simulink model "pasp_16ch_ct"  (Simulink 6.2)
settings: Solver=ode45  StartTime=0.0  StopTime=30000  RelTol=1e-3
undefined symbols (not defined in the file or in its folder): iBOB
libraries: xbsIndex_r3 x1479, casper_library x148, xps_library x58
(part 1 of 11)
settings Model: LastModifiedBy=tfiliba
settings DebuggingCC: SolverPrmCheckMsg=warning

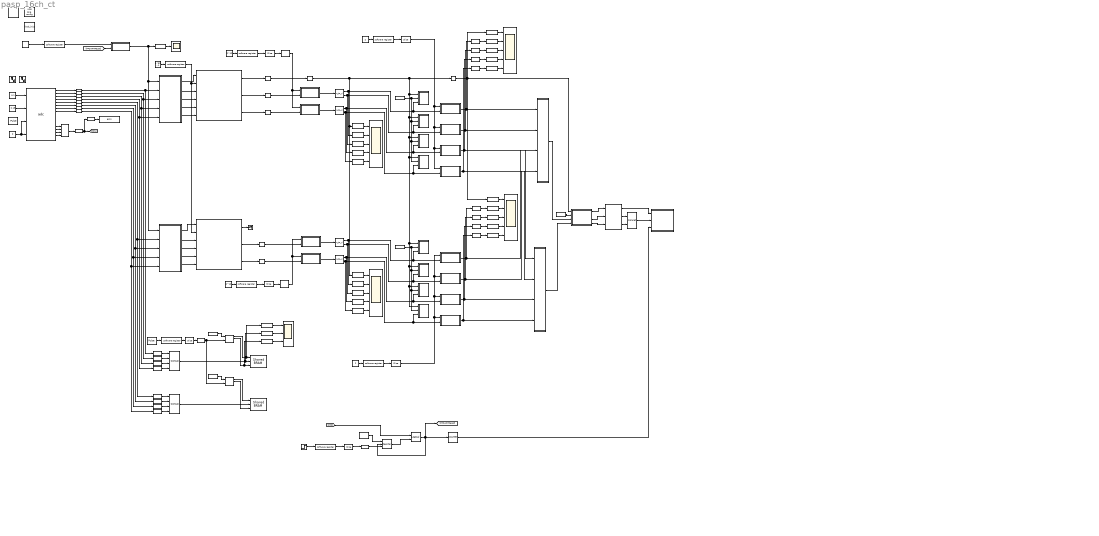
== system pasp_16ch_ct ==
  note: left
  note: Packetized Astronomy Signal Processor
      | Terry Filiba (CASPER)
      | January 2009
      | Version 1.0
  note: n * LCM(reoder_order=2)*(taps*clksperFFT=2*64=128)=256
  note: Pol 1
  note: Pol 2
  note: Real sampling at 800MSa/sec
      | to give B/W of 0-400MHz
  note: ADC Scope
      | Outputs raw bits from ADC so you can measure voltage levels
  note: ARM/PPS Reset Circuit
      | 1. User sets ARM high at half-second
      | 2. 1PPS arrives.
      | 3. PPSARMReset signal goes high for one clock on the 1PPS
      | 4. ARM is reset, and won't go high again until user brings it low then high
  note: Unsigned, 18-bits, b.p. at 12
      | Coefficient by which to scale the output of the FFT.
  note: Selects which 8 bits from 18 are outputted.
      | 0 is lowest 8-bits: bits 0-7 (inclusive)
      | 1: bits 4-9
      | 2: bits 8-15
      | 3 is highest 8-bits: bits 10-17
  note: Extract 8 bits from 18
  note: Extract 8 bits from 18
  note: Delay is here for timing purposes:
      | otherwise adc_sync fails timing.
  " System Generator" : xbsIndex_r3/ System Generator  Tag=genX  xilinxfamily=Virtex2P  part=xc2vp50  speed=-7  package=ff1152  synthesis_tool=XST  directory=./nancay_16ch_ct/sysgen  testbench=off  simulink_period=1  sysclk_period=5  incr_netlist=off  trim_vbits=Everywhere in SubSystem  dbl_ovrd=According to Block Masks  core_generation=According to Block Masks  run_coregen=off  deprecated_control=off  eval_field=0
      settings: AttributesFormatString=System\nGenerator
  Concat1 : xbsIndex_r3/Concat  num_inputs=2  explicit_period=off  period=1  dbl_ovrd=off
  Constant2 : Constant  Value=2
  Constant3 : Constant  Value=2^12
  Constant4 : Constant  Value=2^12
  Constant5 : Constant  Value=2^32 - 1
  Constant6 : Constant  Value=2
  Gateway Out{1..3,8,10..19,21..30} (24 alike) : xbsIndex_r3/Gateway Out  output_type=Double  nbits=8  bin_pt=6  arith_type=Boolean  quantization=Truncate  overflow=Wrap  hdl_port=on  timing_constraint=None  locs_specified=off  LOCs={}  needs_fixed_name=off  show_param=off
      settings: xl_area=[0, 0, 0, 0, 0, 0, 0]
  Reinterpret{,1..3,8..11} (8 alike) : xbsIndex_r3/Reinterpret  force_arith_type=on  arith_type="Signed  (2's comp)"  force_bin_pt=on  bin_pt=0  force_valid=on
  Scope : Scope  NumInputPorts=3
      settings: YMin=-5~-5~-5  YMax=5~5~5
  Scope2 : Scope
      settings: YMin=-1  YMax=1  SaveName=ScopeData2
  Scope{3..6} (4 alike) : Scope  NumInputPorts=5
      Scope3 settings: YMin=-1~-2.5e-005~-1.75e-005~-2.5e-005~-8e-006  YMax=1~0~0~0~0  SaveName=ScopeData3
      Scope4 settings: YMin=-1~-1~-1~-1~-1  YMax=1~0~0~0~0  SaveName=ScopeData4
      Scope5 settings: YMin=-1~-2.5e-005~-1.75e-005~-2.5e-005~-8e-006  YMax=1~0~0~0~0  SaveName=ScopeData5
      Scope6 settings: YMin=-1~-1~-1~-1~-1  YMax=1~0~0~0~0  SaveName=ScopeData6
  Slice10 : xbsIndex_r3/Slice  mode=Lower Bit Location + Width  nbits=2  bit1=0  base1=MSB of Input  bit0=0  base0=LSB of Input  boolean_output=off  explicit_period=off  period=1  dbl_ovrd=off
  Slice2 : xbsIndex_r3/Slice  mode=Lower Bit Location + Width  nbits=2  bit1=0  base1=MSB of Input  bit0=0  base0=LSB of Input  boolean_output=off  explicit_period=off  period=1  dbl_ovrd=off
  Slice3 : xbsIndex_r3/Slice  mode=Lower Bit Location + Width  nbits=18  bit1=0  base1=MSB of Input  bit0=0  base0=LSB of Input  boolean_output=off  explicit_period=off  period=1  dbl_ovrd=off
  Slice4 : xbsIndex_r3/Slice  mode=Lower Bit Location + Width  nbits=18  bit1=0  base1=MSB of Input  bit0=0  base0=LSB of Input  boolean_output=off  explicit_period=off  period=1  dbl_ovrd=off
  Slice8 : xbsIndex_r3/Slice  mode=Lower Bit Location + Width  nbits=1  bit1=0  base1=MSB of Input  bit0=0  base0=LSB of Input  boolean_output=on  explicit_period=off  period=1  dbl_ovrd=off
  Terminator : Terminator
  XSG core config : xps_library/XSG core config  Tag=xps:xsg  hw_sys=iBOB  ibob_linux=off  clk_src=adc1_clk  gpio_clk_io_group=iBOB:sma  gpio_clk_bit_index=0  clk_rate=200  sample_period=1  synthesis_tool=XST  mpc_type=powerpc405
  adc : xps_library/adc  Tag=xps:adc  adc_brd=iBOB:adc1  adc_clk_rate=800  adc_interleave=off  sample_period=1
  adc_data_delay{1..8} (8 alike) : xbsIndex_r3/Delay  latency=1  reg_retiming=on  explicit_period=off  period=1  en=off  accept_only_valid=off  init_zero=on  dbl_ovrd=off  show_param=off
      settings: xl_area=[0, 0, 0, 0, 0, 0, 0]
  bitselect_1 : Subsystem
  bitselect_2 : Subsystem
  bitselect_3 : Subsystem
  bitselect_4 : Subsystem
  bitselect_5 : Subsystem
  bitselect_6 : Subsystem
  bitselect_7 : Subsystem
  bitselect_8 : Subsystem
  bram_adcscope_1 : xps_library/Shared BRAM  Tag=xps:bram  arith_type="Signed  (2's comp)"  addr_width=11  data_width=32  data_bin_pt=0  init_vals=[1:2^11]  sample_rate=1
  bram_adcscope_2 : xps_library/Shared BRAM  Tag=xps:bram  arith_type="Signed  (2's comp)"  addr_width=11  data_width=32  data_bin_pt=0  init_vals=[1:2^11]  sample_rate=1
  bs_delay : xbsIndex_r3/Delay  latency=1  reg_retiming=off  explicit_period=off  period=1  en=off  accept_only_valid=off  init_zero=on  dbl_ovrd=off  show_param=off
      settings: xl_area=[0, 0, 0, 0, 0, 0, 0]
  c_to_ri{1..4} (4 alike) : casper_library/Misc/c_to_ri  n_bits=18  bin_pt=17
      settings: AttributesFormatString=18_17 r/i
  cns_adcscope_1 : xbsIndex_r3/Constant  const=1  equ=P=C  arith_type=Boolean  n_bits=1  bin_pt=0  opselect=C  inp2=PCIN>>17  opr=+  inp1=P  carry=CIN  iostate=0  explicit_period=on  period=1  dbl_ovrd=off
  cns_adcscope_2 : xbsIndex_r3/Constant  const=1  equ=P=C  arith_type=Boolean  n_bits=1  bin_pt=0  opselect=C  inp2=PCIN>>17  opr=+  inp1=P  carry=CIN  iostate=0  explicit_period=on  period=1  dbl_ovrd=off
  cns_reset : xbsIndex_r3/Constant  const=1  equ=P=C  arith_type=Boolean  n_bits=1  bin_pt=0  opselect=C  inp2=PCIN>>17  opr=+  inp1=P  carry=CIN  iostate=0  explicit_period=on  period=1  dbl_ovrd=off
  cns_scopes_en0 : xbsIndex_r3/Constant  const=1  equ=P=C  arith_type=Boolean  n_bits=1  bin_pt=0  opselect=C  inp2=PCIN>>17  opr=+  inp1=P  carry=CIN  iostate=0  explicit_period=on  period=1  dbl_ovrd=off
  cns_scopes_en1 : xbsIndex_r3/Constant  const=1  equ=P=C  arith_type=Boolean  n_bits=1  bin_pt=0  opselect=C  inp2=PCIN>>17  opr=+  inp1=P  carry=CIN  iostate=0  explicit_period=on  period=1  dbl_ovrd=off
  cns_sync_period : Constant  Value=10240
  cns_trotfrt_rnf2 : xbsIndex_r3/Constant  const=1  equ=P=C  arith_type=Boolean  n_bits=1  bin_pt=0  opselect=C  inp2=PCIN>>17  opr=+  inp1=P  carry=CIN  iostate=0  explicit_period=on  period=1  dbl_ovrd=off
  cnt_adcscope_1 : casper_library/Misc/freeze_cntr  CounterBits=11
  cnt_adcscope_2 : casper_library/Misc/freeze_cntr  CounterBits=11
  coeff_delay : xbsIndex_r3/Delay  latency=6  reg_retiming=on  explicit_period=off  period=1  en=off  accept_only_valid=off  init_zero=on  dbl_ovrd=off  show_param=off
      settings: xl_area=[0, 0, 0, 0, 0, 0, 0]
  concat_adcscope_1 : xbsIndex_r3/Concat  num_inputs=4  explicit_period=off  period=1  dbl_ovrd=off
  concat_adcscope_2 : xbsIndex_r3/Concat  num_inputs=4  explicit_period=off  period=1  dbl_ovrd=off
  cram0 : Subsystem  AncestorBlock=gavrt_library/cram  mask(cram){num_slice=4}
      mask prompts: num_slice "Number of slices"
      mask help: Concatenates inputs together after forcing binary point to zero.
      mask init:
      | cram_init(gcb, ...
      |     'num_slice', num_slice);
  cram1 : Subsystem  AncestorBlock=gavrt_library/cram  mask(cram){num_slice=4}
      mask prompts: num_slice "Number of slices"
      mask help: Concatenates inputs together after forcing binary point to zero.
      mask init:
      | cram_init(gcb, ...
      |     'num_slice', num_slice);
  dist_gbe : Subsystem  mask(dist_gbe){numcomputers=16, numsamples=16, samplesperpacket=64}
      mask prompts: numcomputers "Num IPs (Must be power of 2)"; numsamples "Samples per spectrum (Number of clock cycles to generate 1 spectrum)"; samplesperpacket "Samples per packet (Number of samples to put in a packet)"
      mask init:
      | dist_gbe_init(gcb,...
      |     'numcomputers', numcomputers,...
      |     'numsamples', numsamples,...
      |     'samplesperpacket', samplesperpacket)
      settings: AttributesFormatString=IPs=16
  fft_delay : xbsIndex_r3/Delay  latency=4  reg_retiming=off  explicit_period=off  period=1  en=off  accept_only_valid=off  init_zero=on  dbl_ovrd=off  show_param=off
      settings: xl_area=[0, 0, 0, 0, 0, 0, 0]
  fft_wideband_real : Subsystem  AncestorBlock=casper_library/FFTs/fft_wideband_real  mask(fft_wideband_real){FFTSize=5, BitWidth=18, n_inputs=2, quantization=Truncate, overflow=Wrap, add_latency=2, mult_latency=3, bram_latency=2}
      mask prompts: FFTSize "Size of FFT: (2^?)"; BitWidth "Bit Width"; n_inputs "Number of Simultaneous Inputs: (2^?)"; quantization "Quantization Behavior"; overflow "Overflow Behavior"; add_latency "Add Latency"; mult_latency "Mult Latency"; bram_latency "BRAM Latency"
      mask init:
      | fft_wideband_real_init(gcb,...
      |     'FFTSize', FFTSize,...
      |     'BitWidth', BitWidth,...
      |     'n_inputs', n_inputs,...
      |     'quantization', quantization,...
      |     'overflow', overflow,...
      |     'add_latency', add_latency,...
      |     'mult_latency', mult_latency,...
      |     'bram_latency', bram_latency);
      settings: AttributesFormatString=FFTSize=5, n_inputs=2
      mask StyleString: edit,edit,edit,popup(Truncate|Round  (unbiased: +/- Inf)|Round  (unbiased: Even Values)),popup(Wrap|Saturate|Error),edit,edit,edit
  fft_wideband_real1 : Subsystem  AncestorBlock=casper_library/FFTs/fft_wideband_real  mask(fft_wideband_real){FFTSize=5, BitWidth=18, n_inputs=2, quantization=Truncate, overflow=Wrap, add_latency=2, mult_latency=3, bram_latency=2}
      mask prompts: FFTSize "Size of FFT: (2^?)"; BitWidth "Bit Width"; n_inputs "Number of Simultaneous Inputs: (2^?)"; quantization "Quantization Behavior"; overflow "Overflow Behavior"; add_latency "Add Latency"; mult_latency "Mult Latency"; bram_latency "BRAM Latency"
      mask init: same as pasp_16ch_ct/fft_wideband_real
      settings: AttributesFormatString=FFTSize=5, n_inputs=2
      mask StyleString: edit,edit,edit,popup(Truncate|Round  (unbiased: +/- Inf)|Round  (unbiased: Even Values)),popup(Wrap|Saturate|Error),edit,edit,edit
  fftdata_delay{1..4} (4 alike) : xbsIndex_r3/Delay  latency=4  reg_retiming=on  explicit_period=off  period=1  en=off  accept_only_valid=off  init_zero=on  dbl_ovrd=off  show_param=off
      settings: xl_area=[0, 0, 0, 0, 0, 0, 0]
  force_adc_i{0..7} (8 alike) : xbsIndex_r3/Reinterpret  force_arith_type=on  arith_type=Unsigned  force_bin_pt=on  bin_pt=0  force_valid=on
  ibob_lwip : xps_library/ibob_lwip
  led2_pps : xps_library/gpio  Tag=xps:gpio  io_group=iBOB:led  io_dir=out  arith_type=Boolean  bitwidth=1  bin_pt=0  bit_index=3  sample_period=1  use_single_ended=off  use_ddr=off  reg_iob=on  reg_clk_phase=0  termination=None
  log_arm_pps : xbsIndex_r3/Logical  logical_function=AND  inputs=2  precision=Full  arith_type=Unsigned  n_bits=8  bin_pt=2  align_bp=on  latency=0  explicit_period=off  period=1  en=off  dbl_ovrd=off  show_param=off
      settings: xl_area=[0, 0, 0, 0, 0, 0, 0]
  pfb_fir_real : Subsystem  AncestorBlock=casper_library/PFBs/pfb_fir_real  mask(pfb_fir_real){PFBSize=5, TotalTaps=2, WindowType=hamming, n_inputs=2, MakeBiplex=0, BitWidthIn=8, BitWidthOut=18, CoeffBitWidth=8, CoeffDistMem=1, CoeffRound=0, add_latency=1, mult_latency=2, bram_latency=2, quantization=Truncate, fwidth=1}
      mask prompts: PFBSize "Size of PFB: (2^? pnts)"; TotalTaps "Total Number of Taps:"; WindowType "Windowing Function:"; n_inputs "Number of Simultaneous Inputs: (2^?)"; MakeBiplex "Make Biplex"; BitWidthIn "Input Bitwidth:"; BitWidthOut "Output Bitwidth:"; CoeffBitWidth "Coefficient Bitwidth:"; CoeffDistMem "Use Distributed Memory for Coeffs"; CoeffRound "Round Coefficients"; add_latency "Add Latency"; mult_latency "Mult Latency"; bram_latency "BRAM Latency"; quantization "Quantization Behavior"; fwidth "Bin Width Scaling (normal=1)"
      mask init:
      | pfb_fir_real_init(gcb,...
      |     'PFBSize', PFBSize,...
      |     'TotalTaps', TotalTaps,...
      |     'WindowType', WindowType,...
      |     'n_inputs', n_inputs,...
      |     'MakeBiplex', MakeBiplex,...
      |     'BitWidthIn', BitWidthIn,...
      |     'BitWidthOut', BitWidthOut,...
      |     'CoeffBitWidth', CoeffBitWidth,...
      |     'CoeffDistMem', CoeffDistMem,...
      |     'CoeffRound', CoeffRound,...
      |     'add_latency', add_latency,...
      |     'mult_latency', mult_latency,...
      |     'bram_latency', bram_latency,...
      |     'quantization', quantization,...
      |     'fwidth', fwidth);
      settings: AttributesFormatString=taps=2, add_latency=1
      mask StyleString: edit,edit,popup(bartlett|barthannwin|blackman|blackmanharris|bohamwin|chebwin|flattopwin|gausswin|hamming|hann|kaiser|nuttallwin|parzenwin|rectwin|tukeywin|triang),edit,edit,edit,edit,edit,edit,edit,edit,edit,edit,popup(Truncate|Round  (unbiased: +/- Inf)|Round  (unbiased: Even Values)),edit
  pfb_fir_real1 : Subsystem  AncestorBlock=casper_library/PFBs/pfb_fir_real  mask(pfb_fir_real){PFBSize=5, TotalTaps=3, WindowType=hamming, n_inputs=2, MakeBiplex=0, BitWidthIn=8, BitWidthOut=18, CoeffBitWidth=8, CoeffDistMem=1, CoeffRound=0, add_latency=1, mult_latency=2, bram_latency=2, quantization=Truncate, fwidth=1}
      mask prompts: PFBSize "Size of PFB: (2^? pnts)"; TotalTaps "Total Number of Taps:"; WindowType "Windowing Function:"; n_inputs "Number of Simultaneous Inputs: (2^?)"; MakeBiplex "Make Biplex"; BitWidthIn "Input Bitwidth:"; BitWidthOut "Output Bitwidth:"; CoeffBitWidth "Coefficient Bitwidth:"; CoeffDistMem "Use Distributed Memory for Coeffs"; CoeffRound "Round Coefficients"; add_latency "Add Latency"; mult_latency "Mult Latency"; bram_latency "BRAM Latency"; quantization "Quantization Behavior"; fwidth "Bin Width Scaling (normal=1)"
      mask init: same as pasp_16ch_ct/pfb_fir_real
      settings: AttributesFormatString=taps=3, add_latency=1
      mask StyleString: edit,edit,popup(bartlett|barthannwin|blackman|blackmanharris|bohamwin|chebwin|flattopwin|gausswin|hamming|hann|kaiser|nuttallwin|parzenwin|rectwin|tukeywin|triang),edit,edit,edit,edit,edit,edit,edit,edit,edit,edit,popup(Truncate|Round  (unbiased: +/- Inf)|Round  (unbiased: Even Values)),edit
  posedge_adcscope : casper_library/Misc/posedge  Tag=Rising Edge Detector
  posedge_arm : casper_library/Misc/posedge  Tag=Rising Edge Detector
  posedge_pps : casper_library/Misc/posedge  Tag=Rising Edge Detector
  pulse_ext : casper_library/Misc/pulse_ext  pulse_len=10000000
  reg_adcscope_trigger : xps_library/software register  Tag=xps:sw_reg  io_dir=From Processor  arith_type=Unsigned  bitwidth=32  bin_pt=0  sample_period=1  gw_name=pasp_16ch_ct_reg_adcscope_trigger_user_data_out
  reg_arm : xps_library/software register  Tag=xps:sw_reg  io_dir=From Processor  arith_type=Unsigned  bitwidth=32  bin_pt=0  sample_period=1  gw_name=pasp_16ch_ct_reg_arm_user_data_out
  reg_coeff_pol1 : xps_library/software register  Tag=xps:sw_reg  io_dir=From Processor  arith_type=Unsigned  bitwidth=32  bin_pt=0  sample_period=1  gw_name=pasp_16ch_ct_reg_coeff_pol1_user_data_out
  reg_coeff_pol2 : xps_library/software register  Tag=xps:sw_reg  io_dir=From Processor  arith_type=Unsigned  bitwidth=32  bin_pt=0  sample_period=1  gw_name=pasp_16ch_ct_reg_coeff_pol2_user_data_out
  reg_fft_shift : xps_library/software register  Tag=xps:sw_reg  io_dir=From Processor  arith_type=Unsigned  bitwidth=32  bin_pt=0  sample_period=1  gw_name=pasp_16ch_ct_reg_fft_shift_user_data_out
  reg_output_bitselect_pol1 : xps_library/software register  Tag=xps:sw_reg  io_dir=From Processor  arith_type=Unsigned  bitwidth=32  bin_pt=0  sample_period=1  gw_name=pasp_16ch_ct_reg_output_bitselect_pol1_user_data_out
  reg_output_bitselect_pol2 : xps_library/software register  Tag=xps:sw_reg  io_dir=From Processor  arith_type=Unsigned  bitwidth=32  bin_pt=0  sample_period=1  gw_name=pasp_16ch_ct_reg_output_bitselect_pol2_user_data_out
  reg_reset_arm : xbsIndex_r3/Register  init=0  reg_only_valid=off  explicit_period=on  period=1  rst=on  en=on  out_en=off  dbl_ovrd=off  show_param=off
      settings: xl_area=[0, 0, 0, 0, 0, 0, 0]
  reg_sync_period : xps_library/software register  Tag=xps:sw_reg  io_dir=From Processor  arith_type=Unsigned  bitwidth=32  bin_pt=0  sample_period=1  gw_name=pasp_16ch_ct_reg_sync_period_user_data_out
  reint : xbsIndex_r3/Reinterpret  force_arith_type=on  arith_type=Unsigned  force_bin_pt=on  bin_pt=12  force_valid=on
  reint1 : xbsIndex_r3/Reinterpret  force_arith_type=on  arith_type=Unsigned  force_bin_pt=on  bin_pt=12  force_valid=on
  reorder : Subsystem  AncestorBlock=casper_library/Reorder/reorder  mask(reorder){map=[0 8 1 9 2 10 3 11 4 12 5 13 6 14 7 15], n_inputs=2, bram_latency=2, map_latency=1, double_buffer=0}
      mask prompts: map "Output Order:"; n_inputs "Number of inputs"; bram_latency "BRAM Latency"; map_latency "Map Latency"; double_buffer "Double Buffer"
      mask init:
      | reorder_init(gcb, ...
      |     'map', map, ...
      |     'n_inputs', n_inputs, ...
      |     'bram_latency', bram_latency, ...
      |     'map_latency', map_latency, ...
      |     'double_buffer', double_buffer);
      settings: AttributesFormatString=order=4
  scale1 : Subsystem
  scale2 : Subsystem
  scale3 : Subsystem
  scale4 : Subsystem
  scope_output1 : Subsystem
  scope_output2 : Subsystem
  scope_output3 : Subsystem
  scope_output4 : Subsystem
  scope_output5 : Subsystem
  scope_output6 : Subsystem
  scope_output7 : Subsystem
  scope_output8 : Subsystem
  sim_1pps : DiscretePulseGenerator  Period=1000  PulseWidth=3
  sim_adcscope_trigger : DiscretePulseGenerator  Period=5000
  sim_cns : Constant  Value=0.1
  sim_cns1 : Constant  Value=0.15
  sim_sine : Sin  Amplitude=0.8  Frequency=2 * pi * (256/1024)  Samples=0.12566  SampleTime=1/4
  sim_sine1 : Sin  Amplitude=0.8  Frequency=2 * pi * (128/1024)  Samples=0.12566  SampleTime=1/4
  sim_step_arm : Step  SampleTime=0
  sim_zero : Constant  Value=0
  slc_arm : xbsIndex_r3/Slice  mode=Lower Bit Location + Width  nbits=1  bit1=0  base1=MSB of Input  bit0=0  base0=LSB of Input  boolean_output=on  explicit_period=off  period=1  dbl_ovrd=off
  square_transposer : casper_library/Reorder/square_transposer  n_inputs=1
      settings: AttributesFormatString=n_inputs=1
  sync_generator : Subsystem
  sync_or : xbsIndex_r3/Logical  logical_function=OR  inputs=4  precision=Full  arith_type=Unsigned  n_bits=8  bin_pt=2  align_bp=on  latency=1  explicit_period=off  period=1  en=off  dbl_ovrd=off  show_param=off
      settings: xl_area=[0, 0, 0, 0, 0, 0, 0]
  system_counter : xbsIndex_r3/Counter  cnt_type=Free Running  n_bits=64  bin_pt=0  arith_type=Unsigned  start_count=0  cnt_to=Inf  cnt_by_val=1  operation=Up  explicit_period=off  period=1  load_pin=off  rst=on  en=off  dbl_ovrd=off  show_param=off  use_rpm=on  gen_core=off
      settings: xl_area=[0, 0, 0, 0, 0, 0, 0]
  wires:
  reg_fft_shift/1 -> fft_wideband_real/2(shift), fft_wideband_real1/2(shift)
  fft_wideband_real/1(sync_out) -> fft_delay/1
  fft_wideband_real1/1(sync_out) -> Terminator/1
  reg_sync_period/1 -> sync_generator/1(period)
  sim_zero/1 -> adc/4, adc/3
  adc/1 -> adc_data_delay1/1
  sync_generator/1(sync) -> Gateway Out8/1, pfb_fir_real/1(sync), pfb_fir_real1/1(sync)
  adc/2 -> adc_data_delay2/1
  adc/3 -> adc_data_delay3/1
  adc/4 -> adc_data_delay4/1
  adc/5 -> adc_data_delay5/1
  adc/6 -> adc_data_delay6/1
  adc/7 -> adc_data_delay7/1
  adc/8 -> adc_data_delay8/1
  cns_sync_period/1 -> reg_sync_period/1
  adc/13 -> sync_or/1
  adc/14 -> sync_or/2
  adc/15 -> sync_or/3
  adc/16 -> sync_or/4
  sync_or/1 -> posedge_pps/1
  Gateway Out8/1 -> Scope2/1
  posedge_pps/1 -> [PPS], pulse_ext/1
  [PPSARMReset] -> sync_generator/2(reset)
  pulse_ext/1 -> led2_pps/1
  reg_arm/1 -> slc_arm/1
  cns_reset/1 -> reg_reset_arm/1
  reg_reset_arm/1 -> log_arm_pps/2
  [PPS] -> log_arm_pps/1
  log_arm_pps/1 -> reg_reset_arm/2, system_counter/1, [PPSARMReset]
  slc_arm/1 -> posedge_arm/1
  posedge_arm/1 -> reg_reset_arm/3
  concat_adcscope_1/1 -> bram_adcscope_1/2, Gateway Out2/1
  force_adc_i0/1 -> concat_adcscope_1/1
  force_adc_i1/1 -> concat_adcscope_1/2
  force_adc_i2/1 -> concat_adcscope_1/3
  force_adc_i3/1 -> concat_adcscope_1/4
  force_adc_i4/1 -> concat_adcscope_2/1
  force_adc_i5/1 -> concat_adcscope_2/2
  force_adc_i6/1 -> concat_adcscope_2/3
  force_adc_i7/1 -> concat_adcscope_2/4
  sim_step_arm/1 -> reg_arm/1
  Constant3/1 -> reg_coeff_pol1/1
  reg_coeff_pol1/1 -> Slice3/1
  fft_wideband_real/2(out0) -> fftdata_delay1/1
  Slice3/1 -> reint/1
  coeff_delay/1 -> scope_output1/1(rst), scope_output2/1(rst), scope_output3/1(rst), scope_output5/1(rst), scope_output6/1(rst), scope_output7/1(rst), scope_output8/1(rst), scope_output4/1(rst), bs_delay/1, Gateway Out11/1, Gateway Out22/1
  scale1/1(data_out) -> c_to_ri1/1
  reint/1 -> scale1/1(coeff), scale2/1(coeff)
  scale2/1(data_out) -> c_to_ri2/1
  fft_wideband_real/3(out1) -> fftdata_delay2/1
  fft_wideband_real1/2(out0) -> fftdata_delay3/1
  fft_wideband_real1/3(out1) -> fftdata_delay4/1
  Constant4/1 -> reg_coeff_pol2/1
  reg_coeff_pol2/1 -> Slice4/1
  Slice4/1 -> reint1/1
  reint1/1 -> scale3/1(coeff), scale4/1(coeff)
  Constant2/1 -> reg_output_bitselect_pol1/1
  reg_output_bitselect_pol1/1 -> Slice2/1
  c_to_ri1/1 -> bitselect_1/2(data_in), scope_output1/3(data_in), Gateway Out12/1
  c_to_ri2/2 -> Gateway Out14/1, bitselect_4/2(data_in), scope_output4/3(data_in)
  c_to_ri2/1 -> Gateway Out13/1, bitselect_3/2(data_in), scope_output3/3(data_in)
  c_to_ri1/2 -> scope_output2/3(data_in), bitselect_2/2(data_in), Gateway Out10/1
  bitselect_1/1(data_out) -> cram0/1(In1), Reinterpret/1
  bitselect_2/1(data_out) -> cram0/2(In2), Reinterpret1/1
  bitselect_3/1(data_out) -> Reinterpret2/1, cram1/1(In1)
  bitselect_4/1(data_out) -> Reinterpret3/1, cram1/2(In2)
  Constant5/1 -> reg_fft_shift/1
  cnt_adcscope_1/1 -> bram_adcscope_1/1, Gateway Out1/1
  cnt_adcscope_1/2 -> bram_adcscope_1/3, Gateway Out3/1
  cns_adcscope_1/1 -> cnt_adcscope_1/1
  sim_adcscope_trigger/1 -> reg_adcscope_trigger/1
  reg_adcscope_trigger/1 -> Slice8/1
  posedge_adcscope/1 -> cnt_adcscope_1/2, cnt_adcscope_2/2
  concat_adcscope_2/1 -> bram_adcscope_2/2
  cnt_adcscope_2/1 -> bram_adcscope_2/1
  cnt_adcscope_2/2 -> bram_adcscope_2/3
  cns_adcscope_2/1 -> cnt_adcscope_2/1
  Gateway Out1/1 -> Scope/1
  Gateway Out2/1 -> Scope/2
  Gateway Out3/1 -> Scope/3
  cns_scopes_en0/1 -> scope_output1/2(en), scope_output2/2(en), scope_output3/2(en), scope_output4/2(en)
  Slice2/1 -> bitselect_1/1(bitselect), bitselect_2/1(bitselect), bitselect_3/1(bitselect), bitselect_4/1(bitselect)
  sim_cns/1 -> adc/1
  Gateway Out11/1 -> Scope3/1
  Gateway Out12/1 -> Scope3/2
  Gateway Out10/1 -> Scope3/3
  Gateway Out13/1 -> Scope3/4
  Gateway Out14/1 -> Scope3/5
  bs_delay/1 -> Gateway Out16/1, Gateway Out27/1, reorder/1(sync)
  Gateway Out16/1 -> Scope4/1
  Gateway Out17/1 -> Scope4/2
  Gateway Out15/1 -> Scope4/3
  Gateway Out18/1 -> Scope4/4
  Gateway Out19/1 -> Scope4/5
  Slice8/1 -> posedge_adcscope/1
  Reinterpret/1 -> Gateway Out17/1
  Reinterpret1/1 -> Gateway Out15/1
  Reinterpret2/1 -> Gateway Out18/1
  Reinterpret3/1 -> Gateway Out19/1
  c_to_ri3/1 -> bitselect_5/2(data_in), scope_output5/3(data_in), Gateway Out23/1
  c_to_ri4/2 -> Gateway Out25/1, bitselect_8/2(data_in), scope_output8/3(data_in)
  c_to_ri4/1 -> Gateway Out24/1, bitselect_7/2(data_in), scope_output7/3(data_in)
  c_to_ri3/2 -> scope_output6/3(data_in), bitselect_6/2(data_in), Gateway Out21/1
  bitselect_5/1(data_out) -> Reinterpret8/1, cram0/3(In3)
  bitselect_6/1(data_out) -> Reinterpret9/1, cram0/4(In4)
  bitselect_7/1(data_out) -> cram1/3(In3), Reinterpret10/1
  bitselect_8/1(data_out) -> cram1/4(In4), Reinterpret11/1
  cns_scopes_en1/1 -> scope_output5/2(en), scope_output6/2(en), scope_output7/2(en), scope_output8/2(en)
  Gateway Out22/1 -> Scope5/1
  Gateway Out23/1 -> Scope5/2
  Gateway Out21/1 -> Scope5/3
  Gateway Out24/1 -> Scope5/4
  Gateway Out25/1 -> Scope5/5
  scale3/1(data_out) -> c_to_ri3/1
  scale4/1(data_out) -> c_to_ri4/1
  Gateway Out27/1 -> Scope6/1
  Gateway Out28/1 -> Scope6/2
  Gateway Out26/1 -> Scope6/3
  Gateway Out29/1 -> Scope6/4
  Gateway Out30/1 -> Scope6/5
  Reinterpret8/1 -> Gateway Out28/1
  Reinterpret9/1 -> Gateway Out26/1
  Reinterpret10/1 -> Gateway Out29/1
  Reinterpret11/1 -> Gateway Out30/1
  sim_cns1/1 -> adc/2
  Constant6/1 -> reg_output_bitselect_pol2/1
  reg_output_bitselect_pol2/1 -> Slice10/1
  Slice10/1 -> bitselect_5/1(bitselect), bitselect_6/1(bitselect), bitselect_7/1(bitselect), bitselect_8/1(bitselect)
  pfb_fir_real/2(pol1_out1) -> fft_wideband_real/3(in0)
  pfb_fir_real/3(pol1_out2) -> fft_wideband_real/4(in1)
  pfb_fir_real/4(pol1_out3) -> fft_wideband_real/5(in2)
  pfb_fir_real/5(pol1_out4) -> fft_wideband_real/6(in3)
  pfb_fir_real1/2(pol1_out1) -> fft_wideband_real1/3(in0)
  pfb_fir_real1/3(pol1_out2) -> fft_wideband_real1/4(in1)
  pfb_fir_real1/4(pol1_out3) -> fft_wideband_real1/5(in2)
  pfb_fir_real1/5(pol1_out4) -> fft_wideband_real1/6(in3)
  pfb_fir_real/1(sync_out) -> fft_wideband_real/1(sync)
  pfb_fir_real1/1(sync_out) -> fft_wideband_real1/1(sync)
  fft_delay/1 -> coeff_delay/1
  fftdata_delay1/1 -> scale1/2(data_in)
  fftdata_delay2/1 -> scale2/2(data_in)
  fftdata_delay3/1 -> scale3/2(data_in)
  fftdata_delay4/1 -> scale4/2(data_in)
  adc_data_delay1/1 -> force_adc_i0/1, pfb_fir_real/2(pol1_in1)
  adc_data_delay2/1 -> force_adc_i1/1, pfb_fir_real/3(pol1_in2)
  adc_data_delay3/1 -> force_adc_i2/1, pfb_fir_real/4(pol1_in3)
  adc_data_delay4/1 -> force_adc_i3/1, pfb_fir_real/5(pol1_in4)
  adc_data_delay5/1 -> force_adc_i4/1, pfb_fir_real1/2(pol1_in1)
  adc_data_delay6/1 -> force_adc_i5/1, pfb_fir_real1/3(pol1_in2)
  adc_data_delay7/1 -> force_adc_i6/1, pfb_fir_real1/4(pol1_in3)
  adc_data_delay8/1 -> force_adc_i7/1, pfb_fir_real1/5(pol1_in4)
  system_counter/1 -> dist_gbe/3(sys_counter)
  square_transposer/1 -> dist_gbe/1(sync)
  square_transposer/2 -> Concat1/1
  square_transposer/3 -> Concat1/2
  Concat1/1 -> dist_gbe/2(data_in)
  reorder/1(sync_out) -> square_transposer/1
  reorder/3(dout0) -> square_transposer/2
  reorder/4(dout1) -> square_transposer/3
  cns_trotfrt_rnf2/1 -> reorder/2(en)
  cram0/1(Out) -> reorder/3(din0)
  cram1/1(Out) -> reorder/4(din1)

== system pasp_16ch_ct/bitselect_1 ==
  bitselect : Inport  Port=1  LatchInput=off
  data_in : Inport  Port=2  LatchInput=off
  mux_bitselect : xbsIndex_r3/Mux  inputs=4  precision=Full  arith_type="Signed  (2's comp)"  n_bits=8  bin_pt=2  quantization=Truncate  overflow=Wrap  latency=1  explicit_period=off  period=1  en=off  dbl_ovrd=off  show_param=off  mux_type=off  use_rpm=off  gen_core=off
      settings: xl_area=[0, 0, 0, 0, 0, 0, 0]
  reint_bp_0 : xbsIndex_r3/Reinterpret  force_arith_type=on  arith_type=Unsigned  force_bin_pt=on  bin_pt=0  force_valid=on
  slc_bitselect_1 : xbsIndex_r3/Slice  mode=Lower Bit Location + Width  nbits=8  bit1=0  base1=MSB of Input  bit0=0  base0=LSB of Input  boolean_output=off  explicit_period=off  period=1  dbl_ovrd=off
  slc_bitselect_2 : xbsIndex_r3/Slice  mode=Lower Bit Location + Width  nbits=8  bit1=0  base1=MSB of Input  bit0=4  base0=LSB of Input  boolean_output=off  explicit_period=off  period=1  dbl_ovrd=off
  slc_bitselect_3 : xbsIndex_r3/Slice  mode=Lower Bit Location + Width  nbits=8  bit1=0  base1=MSB of Input  bit0=8  base0=LSB of Input  boolean_output=off  explicit_period=off  period=1  dbl_ovrd=off
  slc_bitselect_4 : xbsIndex_r3/Slice  mode=Lower Bit Location + Width  nbits=8  bit1=0  base1=MSB of Input  bit0=10  base0=LSB of Input  boolean_output=off  explicit_period=off  period=1  dbl_ovrd=off
  data_out : Outport
  wires:
  slc_bitselect_1/1 -> mux_bitselect/2
  slc_bitselect_2/1 -> mux_bitselect/3
  slc_bitselect_3/1 -> mux_bitselect/4
  slc_bitselect_4/1 -> mux_bitselect/5
  data_in/1 -> reint_bp_0/1
  bitselect/1 -> mux_bitselect/1
  mux_bitselect/1 -> data_out/1
  reint_bp_0/1 -> slc_bitselect_4/1, slc_bitselect_3/1, slc_bitselect_2/1, slc_bitselect_1/1

== system pasp_16ch_ct/bitselect_2 ==
  bitselect : Inport  Port=1  LatchInput=off
  data_in : Inport  Port=2  LatchInput=off
  mux_bitselect : xbsIndex_r3/Mux  inputs=4  precision=Full  arith_type="Signed  (2's comp)"  n_bits=8  bin_pt=2  quantization=Truncate  overflow=Wrap  latency=1  explicit_period=off  period=1  en=off  dbl_ovrd=off  show_param=off  mux_type=off  use_rpm=off  gen_core=off
      settings: xl_area=[0, 0, 0, 0, 0, 0, 0]
  reint_bp_0 : xbsIndex_r3/Reinterpret  force_arith_type=on  arith_type=Unsigned  force_bin_pt=on  bin_pt=0  force_valid=on
  slc_bitselect_1 : xbsIndex_r3/Slice  mode=Lower Bit Location + Width  nbits=8  bit1=0  base1=MSB of Input  bit0=0  base0=LSB of Input  boolean_output=off  explicit_period=off  period=1  dbl_ovrd=off
  slc_bitselect_2 : xbsIndex_r3/Slice  mode=Lower Bit Location + Width  nbits=8  bit1=0  base1=MSB of Input  bit0=4  base0=LSB of Input  boolean_output=off  explicit_period=off  period=1  dbl_ovrd=off
  slc_bitselect_3 : xbsIndex_r3/Slice  mode=Lower Bit Location + Width  nbits=8  bit1=0  base1=MSB of Input  bit0=8  base0=LSB of Input  boolean_output=off  explicit_period=off  period=1  dbl_ovrd=off
  slc_bitselect_4 : xbsIndex_r3/Slice  mode=Lower Bit Location + Width  nbits=8  bit1=0  base1=MSB of Input  bit0=10  base0=LSB of Input  boolean_output=off  explicit_period=off  period=1  dbl_ovrd=off
  data_out : Outport
  wires:
  reint_bp_0/1 -> slc_bitselect_1/1, slc_bitselect_2/1, slc_bitselect_3/1, slc_bitselect_4/1
  mux_bitselect/1 -> data_out/1
  bitselect/1 -> mux_bitselect/1
  data_in/1 -> reint_bp_0/1
  slc_bitselect_4/1 -> mux_bitselect/5
  slc_bitselect_3/1 -> mux_bitselect/4
  slc_bitselect_2/1 -> mux_bitselect/3
  slc_bitselect_1/1 -> mux_bitselect/2

== system pasp_16ch_ct/bitselect_3 ==
  bitselect : Inport  Port=1  LatchInput=off
  data_in : Inport  Port=2  LatchInput=off
  mux_bitselect : xbsIndex_r3/Mux  inputs=4  precision=Full  arith_type="Signed  (2's comp)"  n_bits=8  bin_pt=2  quantization=Truncate  overflow=Wrap  latency=1  explicit_period=off  period=1  en=off  dbl_ovrd=off  show_param=off  mux_type=off  use_rpm=off  gen_core=off
      settings: xl_area=[0, 0, 0, 0, 0, 0, 0]
  reint_bp_0 : xbsIndex_r3/Reinterpret  force_arith_type=on  arith_type=Unsigned  force_bin_pt=on  bin_pt=0  force_valid=on
  slc_bitselect_1 : xbsIndex_r3/Slice  mode=Lower Bit Location + Width  nbits=8  bit1=0  base1=MSB of Input  bit0=0  base0=LSB of Input  boolean_output=off  explicit_period=off  period=1  dbl_ovrd=off
  slc_bitselect_2 : xbsIndex_r3/Slice  mode=Lower Bit Location + Width  nbits=8  bit1=0  base1=MSB of Input  bit0=4  base0=LSB of Input  boolean_output=off  explicit_period=off  period=1  dbl_ovrd=off
  slc_bitselect_3 : xbsIndex_r3/Slice  mode=Lower Bit Location + Width  nbits=8  bit1=0  base1=MSB of Input  bit0=8  base0=LSB of Input  boolean_output=off  explicit_period=off  period=1  dbl_ovrd=off
  slc_bitselect_4 : xbsIndex_r3/Slice  mode=Lower Bit Location + Width  nbits=8  bit1=0  base1=MSB of Input  bit0=10  base0=LSB of Input  boolean_output=off  explicit_period=off  period=1  dbl_ovrd=off
  data_out : Outport
  wires:
  slc_bitselect_1/1 -> mux_bitselect/2
  slc_bitselect_2/1 -> mux_bitselect/3
  slc_bitselect_3/1 -> mux_bitselect/4
  slc_bitselect_4/1 -> mux_bitselect/5
  data_in/1 -> reint_bp_0/1
  bitselect/1 -> mux_bitselect/1
  mux_bitselect/1 -> data_out/1
  reint_bp_0/1 -> slc_bitselect_4/1, slc_bitselect_3/1, slc_bitselect_2/1, slc_bitselect_1/1

== system pasp_16ch_ct/bitselect_4 ==
  bitselect : Inport  Port=1  LatchInput=off
  data_in : Inport  Port=2  LatchInput=off
  mux_bitselect : xbsIndex_r3/Mux  inputs=4  precision=Full  arith_type="Signed  (2's comp)"  n_bits=8  bin_pt=2  quantization=Truncate  overflow=Wrap  latency=1  explicit_period=off  period=1  en=off  dbl_ovrd=off  show_param=off  mux_type=off  use_rpm=off  gen_core=off
      settings: xl_area=[0, 0, 0, 0, 0, 0, 0]
  reint_bp_0 : xbsIndex_r3/Reinterpret  force_arith_type=on  arith_type=Unsigned  force_bin_pt=on  bin_pt=0  force_valid=on
  slc_bitselect_1 : xbsIndex_r3/Slice  mode=Lower Bit Location + Width  nbits=8  bit1=0  base1=MSB of Input  bit0=0  base0=LSB of Input  boolean_output=off  explicit_period=off  period=1  dbl_ovrd=off
  slc_bitselect_2 : xbsIndex_r3/Slice  mode=Lower Bit Location + Width  nbits=8  bit1=0  base1=MSB of Input  bit0=4  base0=LSB of Input  boolean_output=off  explicit_period=off  period=1  dbl_ovrd=off
  slc_bitselect_3 : xbsIndex_r3/Slice  mode=Lower Bit Location + Width  nbits=8  bit1=0  base1=MSB of Input  bit0=8  base0=LSB of Input  boolean_output=off  explicit_period=off  period=1  dbl_ovrd=off
  slc_bitselect_4 : xbsIndex_r3/Slice  mode=Lower Bit Location + Width  nbits=8  bit1=0  base1=MSB of Input  bit0=10  base0=LSB of Input  boolean_output=off  explicit_period=off  period=1  dbl_ovrd=off
  data_out : Outport
  wires:
  reint_bp_0/1 -> slc_bitselect_1/1, slc_bitselect_2/1, slc_bitselect_3/1, slc_bitselect_4/1
  mux_bitselect/1 -> data_out/1
  bitselect/1 -> mux_bitselect/1
  data_in/1 -> reint_bp_0/1
  slc_bitselect_4/1 -> mux_bitselect/5
  slc_bitselect_3/1 -> mux_bitselect/4
  slc_bitselect_2/1 -> mux_bitselect/3
  slc_bitselect_1/1 -> mux_bitselect/2

== system pasp_16ch_ct/bitselect_5 ==
  bitselect : Inport  Port=1  LatchInput=off
  data_in : Inport  Port=2  LatchInput=off
  mux_bitselect : xbsIndex_r3/Mux  inputs=4  precision=Full  arith_type="Signed  (2's comp)"  n_bits=8  bin_pt=2  quantization=Truncate  overflow=Wrap  latency=1  explicit_period=off  period=1  en=off  dbl_ovrd=off  show_param=off  mux_type=off  use_rpm=off  gen_core=off
      settings: xl_area=[0, 0, 0, 0, 0, 0, 0]
  reint_bp_0 : xbsIndex_r3/Reinterpret  force_arith_type=on  arith_type=Unsigned  force_bin_pt=on  bin_pt=0  force_valid=on
  slc_bitselect_1 : xbsIndex_r3/Slice  mode=Lower Bit Location + Width  nbits=8  bit1=0  base1=MSB of Input  bit0=0  base0=LSB of Input  boolean_output=off  explicit_period=off  period=1  dbl_ovrd=off
  slc_bitselect_2 : xbsIndex_r3/Slice  mode=Lower Bit Location + Width  nbits=8  bit1=0  base1=MSB of Input  bit0=4  base0=LSB of Input  boolean_output=off  explicit_period=off  period=1  dbl_ovrd=off
  slc_bitselect_3 : xbsIndex_r3/Slice  mode=Lower Bit Location + Width  nbits=8  bit1=0  base1=MSB of Input  bit0=8  base0=LSB of Input  boolean_output=off  explicit_period=off  period=1  dbl_ovrd=off
  slc_bitselect_4 : xbsIndex_r3/Slice  mode=Lower Bit Location + Width  nbits=8  bit1=0  base1=MSB of Input  bit0=10  base0=LSB of Input  boolean_output=off  explicit_period=off  period=1  dbl_ovrd=off
  data_out : Outport
  wires:
  slc_bitselect_1/1 -> mux_bitselect/2
  slc_bitselect_2/1 -> mux_bitselect/3
  slc_bitselect_3/1 -> mux_bitselect/4
  slc_bitselect_4/1 -> mux_bitselect/5
  data_in/1 -> reint_bp_0/1
  bitselect/1 -> mux_bitselect/1
  mux_bitselect/1 -> data_out/1
  reint_bp_0/1 -> slc_bitselect_4/1, slc_bitselect_3/1, slc_bitselect_2/1, slc_bitselect_1/1

== system pasp_16ch_ct/bitselect_6 ==
  bitselect : Inport  Port=1  LatchInput=off
  data_in : Inport  Port=2  LatchInput=off
  mux_bitselect : xbsIndex_r3/Mux  inputs=4  precision=Full  arith_type="Signed  (2's comp)"  n_bits=8  bin_pt=2  quantization=Truncate  overflow=Wrap  latency=1  explicit_period=off  period=1  en=off  dbl_ovrd=off  show_param=off  mux_type=off  use_rpm=off  gen_core=off
      settings: xl_area=[0, 0, 0, 0, 0, 0, 0]
  reint_bp_0 : xbsIndex_r3/Reinterpret  force_arith_type=on  arith_type=Unsigned  force_bin_pt=on  bin_pt=0  force_valid=on
  slc_bitselect_1 : xbsIndex_r3/Slice  mode=Lower Bit Location + Width  nbits=8  bit1=0  base1=MSB of Input  bit0=0  base0=LSB of Input  boolean_output=off  explicit_period=off  period=1  dbl_ovrd=off
  slc_bitselect_2 : xbsIndex_r3/Slice  mode=Lower Bit Location + Width  nbits=8  bit1=0  base1=MSB of Input  bit0=4  base0=LSB of Input  boolean_output=off  explicit_period=off  period=1  dbl_ovrd=off
  slc_bitselect_3 : xbsIndex_r3/Slice  mode=Lower Bit Location + Width  nbits=8  bit1=0  base1=MSB of Input  bit0=8  base0=LSB of Input  boolean_output=off  explicit_period=off  period=1  dbl_ovrd=off
  slc_bitselect_4 : xbsIndex_r3/Slice  mode=Lower Bit Location + Width  nbits=8  bit1=0  base1=MSB of Input  bit0=10  base0=LSB of Input  boolean_output=off  explicit_period=off  period=1  dbl_ovrd=off
  data_out : Outport
  wires:
  reint_bp_0/1 -> slc_bitselect_1/1, slc_bitselect_2/1, slc_bitselect_3/1, slc_bitselect_4/1
  mux_bitselect/1 -> data_out/1
  bitselect/1 -> mux_bitselect/1
  data_in/1 -> reint_bp_0/1
  slc_bitselect_4/1 -> mux_bitselect/5
  slc_bitselect_3/1 -> mux_bitselect/4
  slc_bitselect_2/1 -> mux_bitselect/3
  slc_bitselect_1/1 -> mux_bitselect/2

== system pasp_16ch_ct/bitselect_7 ==
  bitselect : Inport  Port=1  LatchInput=off
  data_in : Inport  Port=2  LatchInput=off
  mux_bitselect : xbsIndex_r3/Mux  inputs=4  precision=Full  arith_type="Signed  (2's comp)"  n_bits=8  bin_pt=2  quantization=Truncate  overflow=Wrap  latency=1  explicit_period=off  period=1  en=off  dbl_ovrd=off  show_param=off  mux_type=off  use_rpm=off  gen_core=off
      settings: xl_area=[0, 0, 0, 0, 0, 0, 0]
  reint_bp_0 : xbsIndex_r3/Reinterpret  force_arith_type=on  arith_type=Unsigned  force_bin_pt=on  bin_pt=0  force_valid=on
  slc_bitselect_1 : xbsIndex_r3/Slice  mode=Lower Bit Location + Width  nbits=8  bit1=0  base1=MSB of Input  bit0=0  base0=LSB of Input  boolean_output=off  explicit_period=off  period=1  dbl_ovrd=off
  slc_bitselect_2 : xbsIndex_r3/Slice  mode=Lower Bit Location + Width  nbits=8  bit1=0  base1=MSB of Input  bit0=4  base0=LSB of Input  boolean_output=off  explicit_period=off  period=1  dbl_ovrd=off
  slc_bitselect_3 : xbsIndex_r3/Slice  mode=Lower Bit Location + Width  nbits=8  bit1=0  base1=MSB of Input  bit0=8  base0=LSB of Input  boolean_output=off  explicit_period=off  period=1  dbl_ovrd=off
  slc_bitselect_4 : xbsIndex_r3/Slice  mode=Lower Bit Location + Width  nbits=8  bit1=0  base1=MSB of Input  bit0=10  base0=LSB of Input  boolean_output=off  explicit_period=off  period=1  dbl_ovrd=off
  data_out : Outport
  wires:
  slc_bitselect_1/1 -> mux_bitselect/2
  slc_bitselect_2/1 -> mux_bitselect/3
  slc_bitselect_3/1 -> mux_bitselect/4
  slc_bitselect_4/1 -> mux_bitselect/5
  data_in/1 -> reint_bp_0/1
  bitselect/1 -> mux_bitselect/1
  mux_bitselect/1 -> data_out/1
  reint_bp_0/1 -> slc_bitselect_4/1, slc_bitselect_3/1, slc_bitselect_2/1, slc_bitselect_1/1

== system pasp_16ch_ct/bitselect_8 ==
  bitselect : Inport  Port=1  LatchInput=off
  data_in : Inport  Port=2  LatchInput=off
  mux_bitselect : xbsIndex_r3/Mux  inputs=4  precision=Full  arith_type="Signed  (2's comp)"  n_bits=8  bin_pt=2  quantization=Truncate  overflow=Wrap  latency=1  explicit_period=off  period=1  en=off  dbl_ovrd=off  show_param=off  mux_type=off  use_rpm=off  gen_core=off
      settings: xl_area=[0, 0, 0, 0, 0, 0, 0]
  reint_bp_0 : xbsIndex_r3/Reinterpret  force_arith_type=on  arith_type=Unsigned  force_bin_pt=on  bin_pt=0  force_valid=on
  slc_bitselect_1 : xbsIndex_r3/Slice  mode=Lower Bit Location + Width  nbits=8  bit1=0  base1=MSB of Input  bit0=0  base0=LSB of Input  boolean_output=off  explicit_period=off  period=1  dbl_ovrd=off
  slc_bitselect_2 : xbsIndex_r3/Slice  mode=Lower Bit Location + Width  nbits=8  bit1=0  base1=MSB of Input  bit0=4  base0=LSB of Input  boolean_output=off  explicit_period=off  period=1  dbl_ovrd=off
  slc_bitselect_3 : xbsIndex_r3/Slice  mode=Lower Bit Location + Width  nbits=8  bit1=0  base1=MSB of Input  bit0=8  base0=LSB of Input  boolean_output=off  explicit_period=off  period=1  dbl_ovrd=off
  slc_bitselect_4 : xbsIndex_r3/Slice  mode=Lower Bit Location + Width  nbits=8  bit1=0  base1=MSB of Input  bit0=10  base0=LSB of Input  boolean_output=off  explicit_period=off  period=1  dbl_ovrd=off
  data_out : Outport
  wires:
  reint_bp_0/1 -> slc_bitselect_1/1, slc_bitselect_2/1, slc_bitselect_3/1, slc_bitselect_4/1
  mux_bitselect/1 -> data_out/1
  bitselect/1 -> mux_bitselect/1
  data_in/1 -> reint_bp_0/1
  slc_bitselect_4/1 -> mux_bitselect/5
  slc_bitselect_3/1 -> mux_bitselect/4
  slc_bitselect_2/1 -> mux_bitselect/3
  slc_bitselect_1/1 -> mux_bitselect/2

== system pasp_16ch_ct/cram0 ==
  In1 : Inport  Port=1  LatchInput=off
  In2 : Inport  Port=2  LatchInput=off
  In3 : Inport  Port=3  LatchInput=off
  In4 : Inport  Port=4  LatchInput=off
  Concat : S-Function  AncestorBlock=xbsIndex_r3/Concat  FunctionName=xlconcat  Parameters=sfcn_mwsv__  mask(Xilinx Bus Concatenator){num_inputs=4, explicit_period=off, period=1, dbl_ovrd=off}
      mask prompts: num_inputs "Number of Inputs"; explicit_period "Use Explicit Sample Period"; period "Sample Period  (use -1 to inherit first known input period)"; dbl_ovrd "Override with Doubles"
      mask help: Concatenates two or more inputs. Inputs must be unsigned with binary point at zero.
      mask init:
      | [designRoot, family, part, speed, package, simulinkPeriod, sysclkPeriod, dbl_ovrd, trimVbit] = xlSysgenSettings(gcb,1,1);
      | [bg,fg] = xlcmap('XBlock',dbl_ovrd);
      | iPos = get_param(gcb,'Position');
      | iWidth=iPos(3)-iPos(1); iHeight=iPos(4)-iPos(2);
      | iCx=iWidth/2;
      | iCy=iHeight/2;
      | [logoX, logoY] = xlogo(iPos);
      | 
      | 
      | 
      | 
      | % one time added for param list
      | numInputs = num_inputs + 1;
      | precision0 = 1;
      | latency = 0;
      | dblOvrd = dbl_ovrd;
      | explicitClk = explicit_period;
      | 
      | 
      | % just pass everything to s-function
      | sfcn_mwsv__ = get_param(gcb, 'MaskWSVariables');
      mask Help: eval('xlWeb(xlhtmldoclink(''Concat''))');
      mask StyleString: popup(2|3|4|5|6|7|8|9|10|11|12|13|14|15|16),checkbox,edit,checkbox
      mask CallbackString: |xlMagicCallback||
      mask Display:
      | patch([0 iWidth iWidth 0],[0 0 iHeight iHeight] , bg);
      | patch(logoX,logoY, fg);
      | port_label('input',1,'hi');
      | port_label('input',num_inputs+1,'lo');
      | port_label('output',1,'cat');
      | ;plot([0 0 iWidth iWidth 0], [0 iHeight iHeight 0 0]);
  Reinterp{1..4} (4 alike) : xbsIndex_r3/Reinterpret  force_arith_type=on  arith_type=Unsigned  force_bin_pt=on  bin_pt=0  force_valid=on
  Out : Outport
  wires:
  Reinterp4/1 -> Concat/4
  In4/1 -> Reinterp4/1
  Reinterp3/1 -> Concat/3
  In3/1 -> Reinterp3/1
  Reinterp2/1 -> Concat/2
  In2/1 -> Reinterp2/1
  Reinterp1/1 -> Concat/1
  In1/1 -> Reinterp1/1
  Concat/1 -> Out/1

== system pasp_16ch_ct/cram1 ==
  In1 : Inport  Port=1  LatchInput=off
  In2 : Inport  Port=2  LatchInput=off
  In3 : Inport  Port=3  LatchInput=off
  In4 : Inport  Port=4  LatchInput=off
  Concat : S-Function  AncestorBlock=xbsIndex_r3/Concat  FunctionName=xlconcat  Parameters=sfcn_mwsv__  mask(Xilinx Bus Concatenator){num_inputs=4, explicit_period=off, period=1, dbl_ovrd=off}
      mask prompts: num_inputs "Number of Inputs"; explicit_period "Use Explicit Sample Period"; period "Sample Period  (use -1 to inherit first known input period)"; dbl_ovrd "Override with Doubles"
      mask help: Concatenates two or more inputs. Inputs must be unsigned with binary point at zero.
      mask init: same as pasp_16ch_ct/cram0/Concat
      mask Help: eval('xlWeb(xlhtmldoclink(''Concat''))');
      mask StyleString: popup(2|3|4|5|6|7|8|9|10|11|12|13|14|15|16),checkbox,edit,checkbox
      mask CallbackString: |xlMagicCallback||
      mask Display:
      | patch([0 iWidth iWidth 0],[0 0 iHeight iHeight] , bg);
      | patch(logoX,logoY, fg);
      | port_label('input',1,'hi');
      | port_label('input',num_inputs+1,'lo');
      | port_label('output',1,'cat');
      | ;plot([0 0 iWidth iWidth 0], [0 iHeight iHeight 0 0]);
  Reinterp{1..4} (4 alike) : xbsIndex_r3/Reinterpret  force_arith_type=on  arith_type=Unsigned  force_bin_pt=on  bin_pt=0  force_valid=on
  Out : Outport
  wires:
  Reinterp4/1 -> Concat/4
  In4/1 -> Reinterp4/1
  Reinterp3/1 -> Concat/3
  In3/1 -> Reinterp3/1
  Reinterp2/1 -> Concat/2
  In2/1 -> Reinterp2/1
  Reinterp1/1 -> Concat/1
  In1/1 -> Reinterp1/1
  Concat/1 -> Out/1
